simulink model "fuzzy_logiz_control_diafora_a"  (R2019a)
settings: Solver=VariableStepAuto  StartTime=0.0  StopTime=10.0  RelTol=1e-3
libraries: fuzblock x5
settings Model: Creator=Konstantinos  LastModifiedBy=Konstantinos

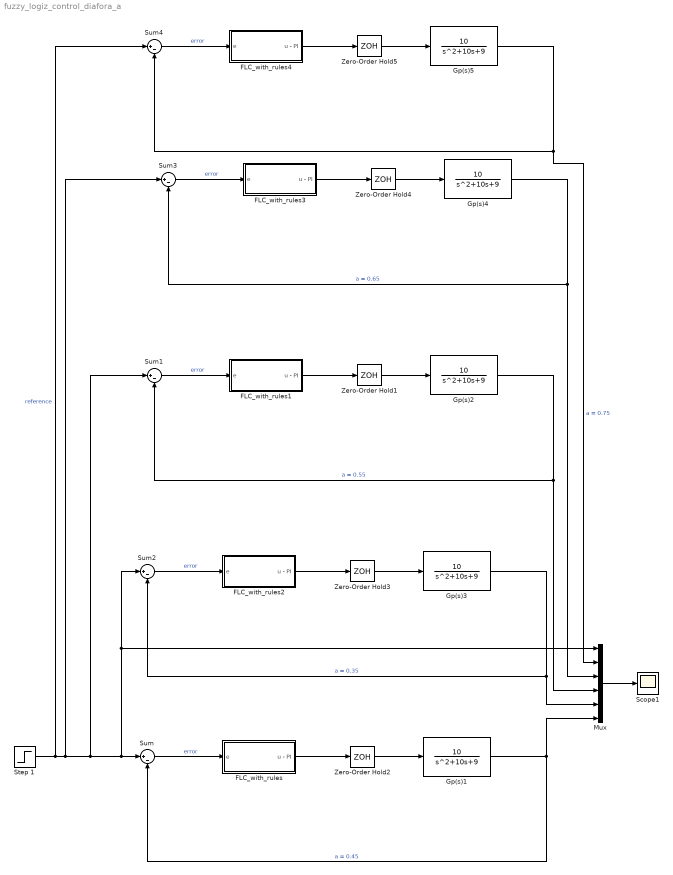
== system fuzzy_logiz_control_diafora_a ==
  FLC_with_rules : Subsystem
  FLC_with_rules1 : Subsystem
  FLC_with_rules2 : Subsystem
  FLC_with_rules3 : Subsystem
  FLC_with_rules4 : Subsystem
  Gp(s){1..5} (5 alike) : TransferFcn  Numerator=[10]  Denominator=[1 10 9]
  Mux : Mux  Inputs=6
  Scope1 : Scope
  Step 1 : Step  Time=0  SampleTime=0.01
  Sum{,1..4} (5 alike) : Sum  Inputs=|+-
  Zero-Order Hold{1..5} (5 alike) : ZeroOrderHold  SampleTime=0.01
  wires:
  FLC_with_rules/1(u - PI) -> Zero-Order Hold2/1
  Zero-Order Hold2/1 -> Gp(s)1/1
  Sum/1 -> FLC_with_rules/1(e)  "error"
  Gp(s)1/1 -> Sum/2, Mux/6  "a = 0.45"
  Mux/1 -> Scope1/1
  Sum1/1 -> FLC_with_rules1/1(e)  "error"
  FLC_with_rules1/1(u - PI) -> Zero-Order Hold1/1
  Zero-Order Hold1/1 -> Gp(s)2/1
  Gp(s)2/1 -> Mux/4, Sum1/2  "a = 0.55"
  Sum2/1 -> FLC_with_rules2/1(e)  "error"
  FLC_with_rules2/1(u - PI) -> Zero-Order Hold3/1
  Zero-Order Hold3/1 -> Gp(s)3/1
  Gp(s)3/1 -> Mux/5, Sum2/2  "a = 0.35"
  Sum3/1 -> FLC_with_rules3/1(e)  "error"
  FLC_with_rules3/1(u - PI) -> Zero-Order Hold4/1
  Zero-Order Hold4/1 -> Gp(s)4/1
  Gp(s)4/1 -> Mux/3, Sum3/2  "a = 0.65"
  Zero-Order Hold5/1 -> Gp(s)5/1
  Step 1/1 -> Sum4/1, Sum3/1, Sum1/1, Sum2/1, Mux/1, Sum/1  "reference"
  Gp(s)5/1 -> Mux/2, Sum4/2  "a = 0.75"
  FLC_with_rules4/1(u - PI) -> Zero-Order Hold5/1
  Sum4/1 -> FLC_with_rules4/1(e)  "error"

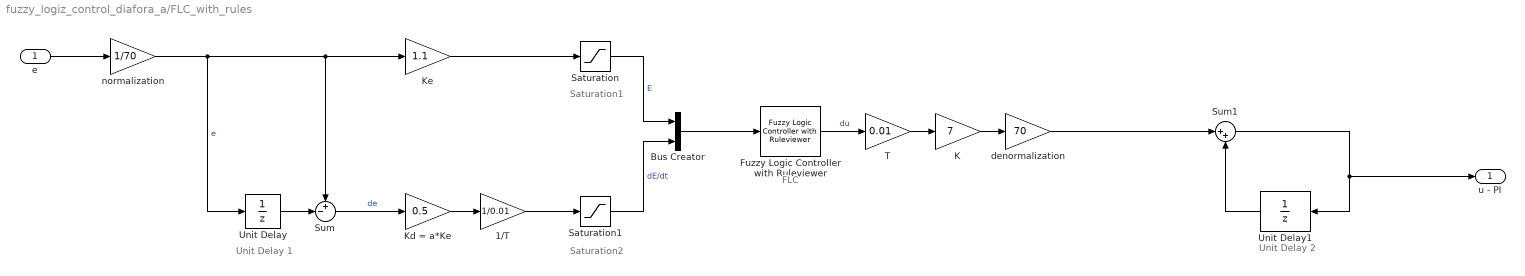
== system fuzzy_logiz_control_diafora_a/FLC_with_rules ==
  note: FLC
  note: Saturation2
  note: Saturation1
  note: Unit Delay 2
  note: Unit Delay 1
  e : Inport
  1/T : Gain  Gain=1/0.01
  Bus Creator : BusCreator  Inputs=2
  Fuzzy Logic Controller with Ruleviewer : fuzblock/Fuzzy Logic  Controller  with Ruleviewer  fismatrix=FLC_with_rules  Ts=0.01
  K : Gain  Gain=7
  Kd = a*Ke : Gain  Gain=0.5
  Ke : Gain  Gain=1.1
  Saturation : Saturate  UpperLimit=1  LowerLimit=-1
  Saturation1 : Saturate  UpperLimit=1  LowerLimit=-1
  Sum : Sum  Inputs=+-|
  Sum1 : Sum  Inputs=|++
  T : Gain  Gain=0.01
  Unit Delay : UnitDelay  SampleTime=-1  HasFrameUpgradeWarning=on
  Unit Delay1 : UnitDelay  SampleTime=-1  HasFrameUpgradeWarning=on
  denormalization : Gain  Gain=70
  normalization : Gain  Gain=1/70
  u - PI : Outport
  wires:
  Sum1/1 -> u - PI/1, Unit Delay1/1
  1/T/1 -> Saturation1/1
  Fuzzy Logic Controller with Ruleviewer/1 -> T/1  "du"
  denormalization/1 -> Sum1/1
  K/1 -> denormalization/1
  Saturation1/1 -> Bus Creator/2  "dE/dt"
  Saturation/1 -> Bus Creator/1  "E"
  Sum/1 -> Kd = a*Ke/1  "de"
  Unit Delay1/1 -> Sum1/2
  normalization/1 -> Ke/1, Sum/1, Unit Delay/1  "e"
  T/1 -> K/1
  Kd = a*Ke/1 -> 1/T/1
  Ke/1 -> Saturation/1
  Unit Delay/1 -> Sum/2
  e/1 -> normalization/1
  Bus Creator/1 -> Fuzzy Logic Controller with Ruleviewer/1

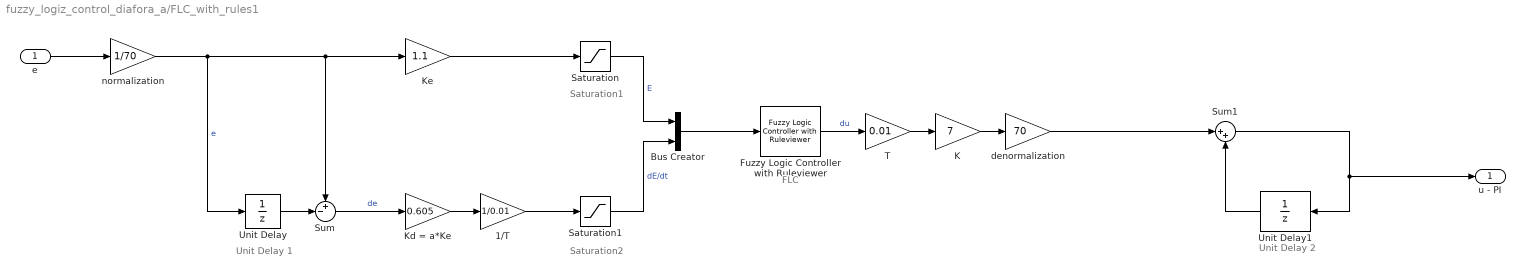
== system fuzzy_logiz_control_diafora_a/FLC_with_rules1 ==
  note: FLC
  note: Saturation2
  note: Saturation1
  note: Unit Delay 2
  note: Unit Delay 1
  e : Inport
  1/T : Gain  Gain=1/0.01
  Bus Creator : BusCreator  Inputs=2
  Fuzzy Logic Controller with Ruleviewer : fuzblock/Fuzzy Logic  Controller  with Ruleviewer  fismatrix=FLC_with_rules  Ts=0.01
  K : Gain  Gain=7
  Kd = a*Ke : Gain  Gain=0.605
  Ke : Gain  Gain=1.1
  Saturation : Saturate  UpperLimit=1  LowerLimit=-1
  Saturation1 : Saturate  UpperLimit=1  LowerLimit=-1
  Sum : Sum  Inputs=+-|
  Sum1 : Sum  Inputs=|++
  T : Gain  Gain=0.01
  Unit Delay : UnitDelay  SampleTime=-1  HasFrameUpgradeWarning=on
  Unit Delay1 : UnitDelay  SampleTime=-1  HasFrameUpgradeWarning=on
  denormalization : Gain  Gain=70
  normalization : Gain  Gain=1/70
  u - PI : Outport
  wires:
  Sum1/1 -> u - PI/1, Unit Delay1/1
  1/T/1 -> Saturation1/1
  Fuzzy Logic Controller with Ruleviewer/1 -> T/1  "du"
  denormalization/1 -> Sum1/1
  K/1 -> denormalization/1
  Saturation1/1 -> Bus Creator/2  "dE/dt"
  Saturation/1 -> Bus Creator/1  "E"
  Sum/1 -> Kd = a*Ke/1  "de"
  Unit Delay1/1 -> Sum1/2
  normalization/1 -> Ke/1, Sum/1, Unit Delay/1  "e"
  T/1 -> K/1
  Kd = a*Ke/1 -> 1/T/1
  Ke/1 -> Saturation/1
  Unit Delay/1 -> Sum/2
  e/1 -> normalization/1
  Bus Creator/1 -> Fuzzy Logic Controller with Ruleviewer/1

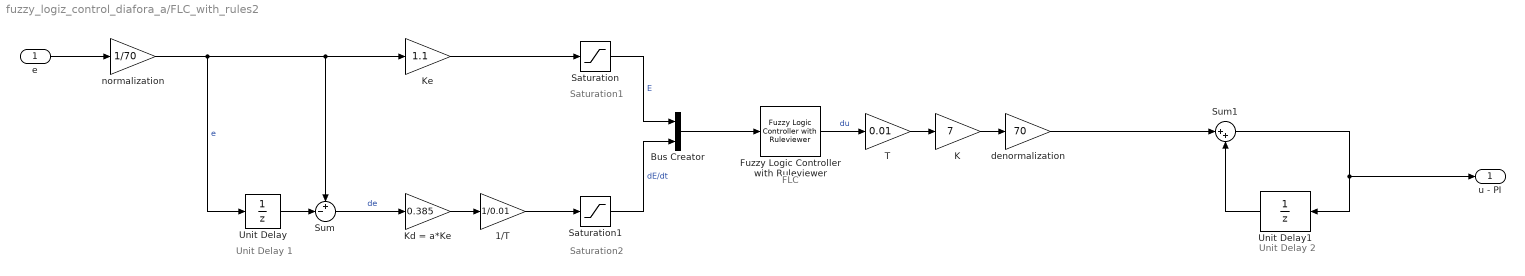
== system fuzzy_logiz_control_diafora_a/FLC_with_rules2 ==
  note: FLC
  note: Saturation2
  note: Saturation1
  note: Unit Delay 2
  note: Unit Delay 1
  e : Inport
  1/T : Gain  Gain=1/0.01
  Bus Creator : BusCreator  Inputs=2
  Fuzzy Logic Controller with Ruleviewer : fuzblock/Fuzzy Logic  Controller  with Ruleviewer  fismatrix=FLC_with_rules  Ts=0.01
  K : Gain  Gain=7
  Kd = a*Ke : Gain  Gain=0.385
  Ke : Gain  Gain=1.1
  Saturation : Saturate  UpperLimit=1  LowerLimit=-1
  Saturation1 : Saturate  UpperLimit=1  LowerLimit=-1
  Sum : Sum  Inputs=+-|
  Sum1 : Sum  Inputs=|++
  T : Gain  Gain=0.01
  Unit Delay : UnitDelay  SampleTime=-1  HasFrameUpgradeWarning=on
  Unit Delay1 : UnitDelay  SampleTime=-1  HasFrameUpgradeWarning=on
  denormalization : Gain  Gain=70
  normalization : Gain  Gain=1/70
  u - PI : Outport
  wires:
  Sum1/1 -> u - PI/1, Unit Delay1/1
  1/T/1 -> Saturation1/1
  Fuzzy Logic Controller with Ruleviewer/1 -> T/1  "du"
  denormalization/1 -> Sum1/1
  K/1 -> denormalization/1
  Saturation1/1 -> Bus Creator/2  "dE/dt"
  Saturation/1 -> Bus Creator/1  "E"
  Sum/1 -> Kd = a*Ke/1  "de"
  Unit Delay1/1 -> Sum1/2
  normalization/1 -> Ke/1, Sum/1, Unit Delay/1  "e"
  T/1 -> K/1
  Kd = a*Ke/1 -> 1/T/1
  Ke/1 -> Saturation/1
  Unit Delay/1 -> Sum/2
  e/1 -> normalization/1
  Bus Creator/1 -> Fuzzy Logic Controller with Ruleviewer/1

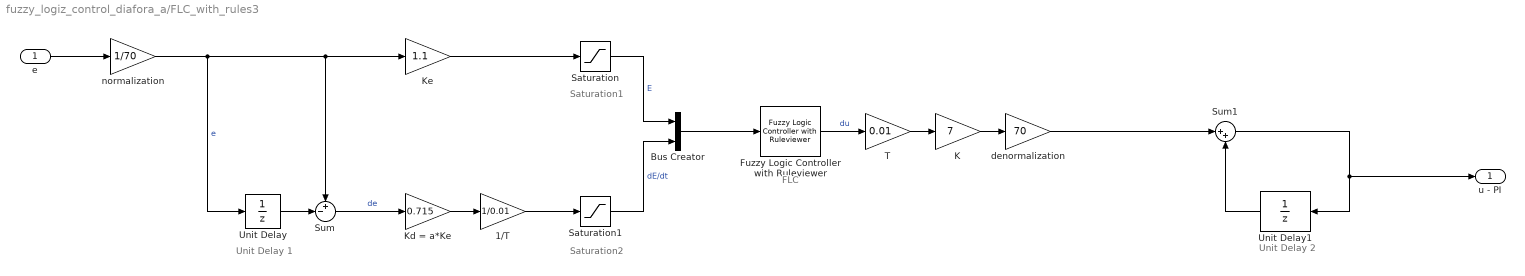
== system fuzzy_logiz_control_diafora_a/FLC_with_rules3 ==
  note: FLC
  note: Saturation2
  note: Saturation1
  note: Unit Delay 2
  note: Unit Delay 1
  e : Inport
  1/T : Gain  Gain=1/0.01
  Bus Creator : BusCreator  Inputs=2
  Fuzzy Logic Controller with Ruleviewer : fuzblock/Fuzzy Logic  Controller  with Ruleviewer  fismatrix=FLC_with_rules  Ts=0.01
  K : Gain  Gain=7
  Kd = a*Ke : Gain  Gain=0.715
  Ke : Gain  Gain=1.1
  Saturation : Saturate  UpperLimit=1  LowerLimit=-1
  Saturation1 : Saturate  UpperLimit=1  LowerLimit=-1
  Sum : Sum  Inputs=+-|
  Sum1 : Sum  Inputs=|++
  T : Gain  Gain=0.01
  Unit Delay : UnitDelay  SampleTime=-1  HasFrameUpgradeWarning=on
  Unit Delay1 : UnitDelay  SampleTime=-1  HasFrameUpgradeWarning=on
  denormalization : Gain  Gain=70
  normalization : Gain  Gain=1/70
  u - PI : Outport
  wires:
  Sum1/1 -> u - PI/1, Unit Delay1/1
  1/T/1 -> Saturation1/1
  Fuzzy Logic Controller with Ruleviewer/1 -> T/1  "du"
  denormalization/1 -> Sum1/1
  K/1 -> denormalization/1
  Saturation1/1 -> Bus Creator/2  "dE/dt"
  Saturation/1 -> Bus Creator/1  "E"
  Sum/1 -> Kd = a*Ke/1  "de"
  Unit Delay1/1 -> Sum1/2
  normalization/1 -> Ke/1, Sum/1, Unit Delay/1  "e"
  T/1 -> K/1
  Kd = a*Ke/1 -> 1/T/1
  Ke/1 -> Saturation/1
  Unit Delay/1 -> Sum/2
  e/1 -> normalization/1
  Bus Creator/1 -> Fuzzy Logic Controller with Ruleviewer/1

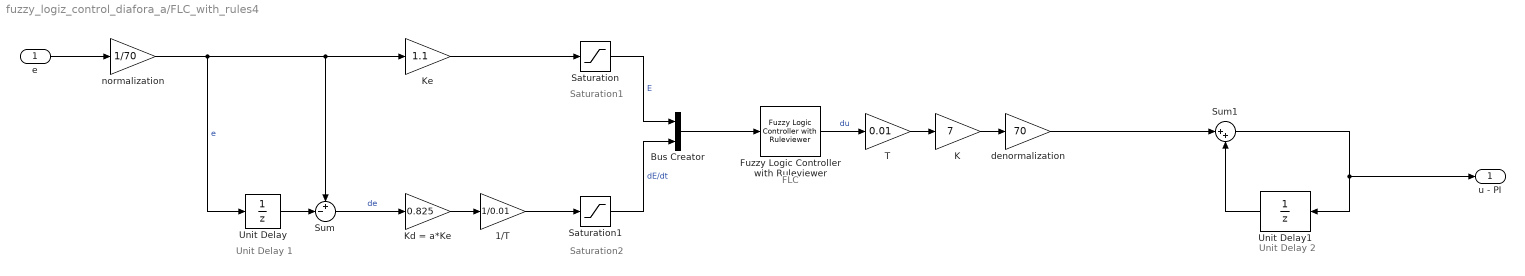
== system fuzzy_logiz_control_diafora_a/FLC_with_rules4 ==
  note: FLC
  note: Saturation2
  note: Saturation1
  note: Unit Delay 2
  note: Unit Delay 1
  e : Inport
  1/T : Gain  Gain=1/0.01
  Bus Creator : BusCreator  Inputs=2
  Fuzzy Logic Controller with Ruleviewer : fuzblock/Fuzzy Logic  Controller  with Ruleviewer  fismatrix=FLC_with_rules  Ts=0.01
  K : Gain  Gain=7
  Kd = a*Ke : Gain  Gain=0.825
  Ke : Gain  Gain=1.1
  Saturation : Saturate  UpperLimit=1  LowerLimit=-1
  Saturation1 : Saturate  UpperLimit=1  LowerLimit=-1
  Sum : Sum  Inputs=+-|
  Sum1 : Sum  Inputs=|++
  T : Gain  Gain=0.01
  Unit Delay : UnitDelay  SampleTime=-1  HasFrameUpgradeWarning=on
  Unit Delay1 : UnitDelay  SampleTime=-1  HasFrameUpgradeWarning=on
  denormalization : Gain  Gain=70
  normalization : Gain  Gain=1/70
  u - PI : Outport
  wires:
  Sum1/1 -> u - PI/1, Unit Delay1/1
  1/T/1 -> Saturation1/1
  Fuzzy Logic Controller with Ruleviewer/1 -> T/1  "du"
  denormalization/1 -> Sum1/1
  K/1 -> denormalization/1
  Saturation1/1 -> Bus Creator/2  "dE/dt"
  Saturation/1 -> Bus Creator/1  "E"
  Sum/1 -> Kd = a*Ke/1  "de"
  Unit Delay1/1 -> Sum1/2
  normalization/1 -> Ke/1, Sum/1, Unit Delay/1  "e"
  T/1 -> K/1
  Kd = a*Ke/1 -> 1/T/1
  Ke/1 -> Saturation/1
  Unit Delay/1 -> Sum/2
  e/1 -> normalization/1
  Bus Creator/1 -> Fuzzy Logic Controller with Ruleviewer/1
